simulink model "ps3"  (R2023a)
settings: Solver=ode4  StartTime=0.0  StopTime=t_duration  FixedStep=dt  MaxStep=max_step_size  RelTol=relative_tolerance
values from neighbouring files (symbols this model uses):
  plant = struct()    [ps3_config.m]
settings Model: Creator=ndelurgio  LastModifiedBy=ndelurgio

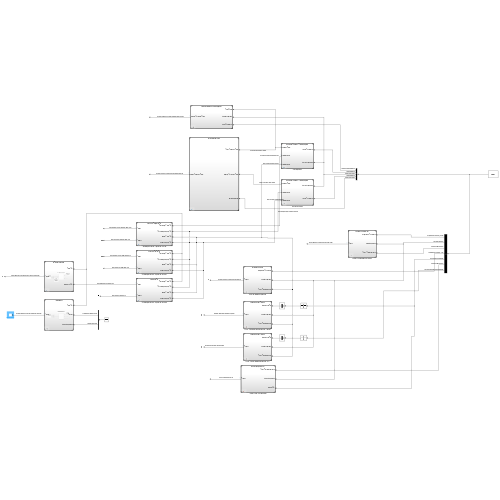
[thumbnail: Simulink's stored preview of the top-level diagram]
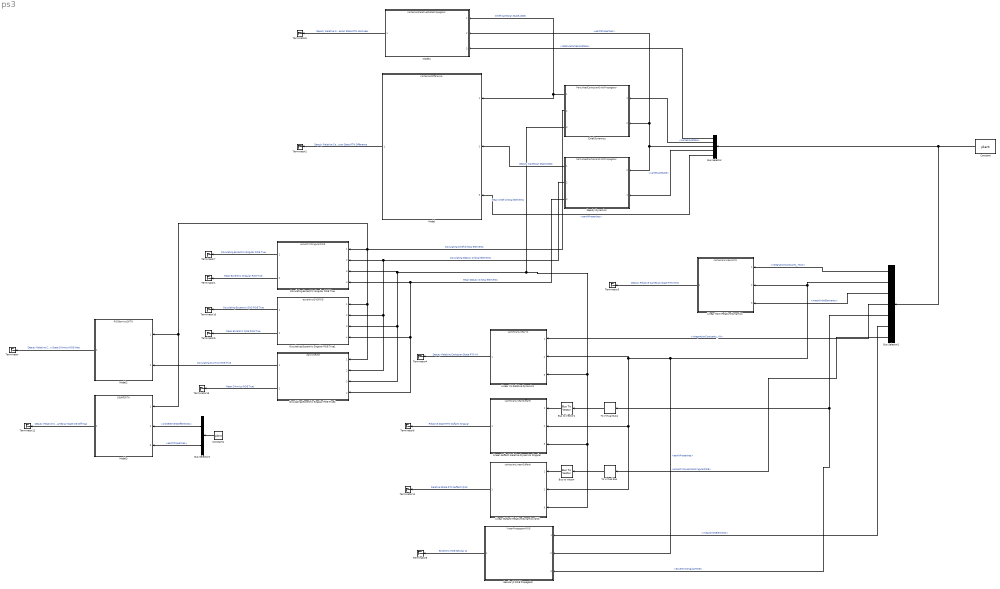
== system ps3 ==
  Bus Selector : BusSelector  OutputSignals=deputy.initialConditions.relativeCartesianState,chief.initialConditions.cartesianState,environment.earthProperties,deputy.initialConditions.cartesianState,environment.earthProperties
  Bus Selector1 : BusSelector  OutputSignals=deputy.initialConditions.integrationConstants_HCW,environment.earthProperties,chief.initialConditions.meanOrbitElements,deputy.initialConditions.integrationConstants_YA,deputy.initialConditions.eccentricSingularROE,chief.initialConditions.meanOrbitElements,deputy.initialConditions.eccentricQuasiNonsingularROE
  Bus Selector2 : BusSelector  OutputSignals=deputy.initialConditions.orbitElementDifferences,environment.earthProperties
  Bus to Vector : BusToVector
  Bus to Vector1 : BusToVector
  Chief Dynamics : ModelReference  ModelNameDialog=PerturbedCartesianOrbitPropagator.slx  SimulationMode=Normal  ModelReferenceVersion=1.136
  Constant : Constant  Value=plant  OutDataTypeStr=Bus: plantBus
  Constant1 : Constant  Value=plant  OutDataTypeStr=Bus: plantBus
  Deputy Dynamics : ModelReference  ModelNameDialog=PerturbedCartesianOrbitPropagator.slx  SimulationMode=Normal  ModelReferenceVersion=1.136
      settings: PortSchema="{\"entries\":[{\"content\":{\"sides\":[{\"content\":{\"connectorIds\":[\"In2\",\"In1\"]},\"type\":\"ConnectorPlacement.EquallySpacedRectSide\",\"uuid\":\"4c211678-740f-40f0-887b-605a3322d7cb\"},{\"content\":{\"connectorIds\":[\"Out1\",\"Out2\",\"Out3\"],\"side\":\"RIGHT\"},\"type\":\"ConnectorPlacement.EquallySpacedRectSide\",\"uuid\":\"7e8d6e44-a7a2-4633-9eac-45eb2a30ed1c\"},{\"content\":{\"side\":\"TOP\"},\"type\":\"ConnectorPlacement.EquallySpacedRectSide\",\"uuid\":\"00358f8f-509c-447f-b607-9e6e4b9aa7b5\"}]},\"type\":\"ConnectorPlacement.EquallySpacedConnector\",\"uuid\":\"f8258235-53bd-4241-8f5f-7f5c3c0a64eb\"}],\"packageUris\":[\"http://schema.mathworks.com/mf0/Connector/R2020b\"],\"version\":\"1.0\"}"
  Linear Guffanti Relative Dynamics QNS : ModelReference  ModelNameDialog=cartesianLinearGuffanti  SimulationMode=Normal  ModelReferenceVersion=1.29
  Linear Guffanti Relative Dynamics Singular : ModelReference  ModelNameDialog=cartesianLinearGuffanti  SimulationMode=Normal  ModelReferenceVersion=1.29
  Linear HCW Relative Dynamics : ModelReference  ModelNameDialog=cartesianLinearHCW  SimulationMode=Normal  ModelReferenceVersion=1.11
  Linear YA Relative Dynamics : ModelReference  ModelNameDialog=cartesianLinearYA  SimulationMode=Normal  ModelReferenceVersion=1.23
  Model : ModelReference  ModelNameDialog=cartesianDifference  SimulationMode=Normal  ModelReferenceVersion=1.33
  Model1 : ModelReference  ModelNameDialog=cartesianRelativeStatePropagator  SimulationMode=Normal  ModelReferenceVersion=1.41
  Model2 : ModelReference  ModelNameDialog=ROEdamico2RTN  SimulationMode=Normal  ModelReferenceVersion=1.9
  Model3 : ModelReference  ModelNameDialog=OEdiff2RTN  SimulationMode=Normal  ModelReferenceVersion=1.12
  Osculating Eccentric Singular ROE True : ModelReference  ModelNameDialog=eccentricSingularROE  SimulationMode=Normal  ModelReferenceVersion=1.13
  Osculating Eccentric Singular ROE True1 : ModelReference  ModelNameDialog=eccentricQNSROE  SimulationMode=Normal  ModelReferenceVersion=1.16
  Osculating Eccentric Singular ROE True2 : ModelReference  ModelNameDialog=damicoROE  SimulationMode=Normal  ModelReferenceVersion=1.17
  Secular J2 ROE Propagator : ModelReference  ModelNameDialog=linearPropagatorROE  SimulationMode=Normal  ModelReferenceVersion=1.11
  Terminator{,1..13} (14 alike) : Terminator
  To Virtual Bus : SignalConversion  ConversionOutput=Virtual bus  OverrideOpt=off
  To Virtual Bus1 : SignalConversion  ConversionOutput=Virtual bus  OverrideOpt=off
  wires:
  Constant/1 -> Bus Selector/1, Bus Selector1/1
  Bus Selector/3 -> Model1/2, Chief Dynamics/2, Deputy Dynamics/2  "<earthProperties>"
  Bus Selector/2 -> Chief Dynamics/1  "<cartesianState>"
  Bus Selector/4 -> Deputy Dynamics/1  "<cartesianState>"
  Chief Dynamics/1 -> Model/1, Model1/1  "Chief Cartesian State J2000"
  Deputy Dynamics/1 -> Model/2  "Deputy Cartesian State J2000"
  Chief Dynamics/2 -> Osculating Eccentric Singular ROE True2/1, Osculating Eccentric Singular ROE True1/1, Model3/1, Model2/1, Osculating Eccentric Singular ROE True/1  "Osculating Chief Orbital Elements"
  Deputy Dynamics/2 -> Osculating Eccentric Singular ROE True2/2, Osculating Eccentric Singular ROE True1/2, Osculating Eccentric Singular ROE True/2  "Osculating Deputy Orbital Elements"
  Bus Selector/5 -> Model/3  "<earthProperties>"
  Model/1 -> Terminator2/1  "Deputy Relative Cartesian State RTN Difference"
  Bus Selector1/3 -> Linear HCW Relative Dynamics/3  "<meanOrbitElements>"
  Bus Selector1/2 -> Secular J2 ROE Propagator/2, Linear Guffanti Relative Dynamics QNS/2, Linear Guffanti Relative Dynamics Singular/2, Linear YA Relative Dynamics/2, Linear HCW Relative Dynamics/2  "<earthProperties>"
  Bus Selector1/1 -> Linear HCW Relative Dynamics/1  "<integrationConstants_HCW>"
  Linear HCW Relative Dynamics/1 -> Terminator3/1  "Deputy Relative Cartesian State RTN HCW"
  Bus Selector/1 -> Model1/3  "<relativeCartesianState>"
  Linear YA Relative Dynamics/1 -> Terminator4/1  "Deputy Relative Cartesian State RTN YA"
  Bus Selector1/4 -> Linear YA Relative Dynamics/1  "<integrationConstants_YA>"
  Model1/1 -> Terminator5/1  "Deputy Relative Cartesian State RTN Nonlinear"
  Linear Guffanti Relative Dynamics Singular/1 -> Terminator6/1  "Relative State RTN Guffanti Singular"
  Bus Selector1/5 -> Secular J2 ROE Propagator/3, To Virtual Bus1/1  "<eccentricSingularROE>"
  Osculating Eccentric Singular ROE True/1 -> Terminator7/1  "Osculating Eccentric Singular ROE True"
  Secular J2 ROE Propagator/1 -> Terminator8/1  "Eccentric ROE Secular J2"
  Bus Selector1/6 -> Secular J2 ROE Propagator/1  "<meanOrbitElements>"
  Chief Dynamics/3 -> Linear Guffanti Relative Dynamics QNS/3, Linear Guffanti Relative Dynamics Singular/3, Linear YA Relative Dynamics/3, Osculating Eccentric Singular ROE True/3, Osculating Eccentric Singular ROE True2/3, Osculating Eccentric Singular ROE True1/3  "Mean Chief Orbital Elements"
  Deputy Dynamics/3 -> Osculating Eccentric Singular ROE True2/4, Osculating Eccentric Singular ROE True1/4, Osculating Eccentric Singular ROE True/4  "Mean Deputy Orbital Elements"
  Osculating Eccentric Singular ROE True/2 -> Terminator1/1  "Mean Eccentric Singular ROE True"
  Osculating Eccentric Singular ROE True1/1 -> Terminator10/1  "Osculating Eccentric QNS ROE True"
  Osculating Eccentric Singular ROE True1/2 -> Terminator9/1  "Mean Eccentric QNS ROE True"
  Linear Guffanti Relative Dynamics QNS/1 -> Terminator11/1  "Relative State RTN Guffanti QNS"
  Bus Selector1/7 -> To Virtual Bus/1  "<eccentricQuasiNonsingularROE>"
  Bus to Vector/1 -> Linear Guffanti Relative Dynamics QNS/1
  Bus to Vector1/1 -> Linear Guffanti Relative Dynamics Singular/1
  To Virtual Bus/1 -> Bus to Vector/1
  To Virtual Bus1/1 -> Bus to Vector1/1
  Osculating Eccentric Singular ROE True2/1 -> Model2/2  "Osculating D'Amico ROE True"
  Osculating Eccentric Singular ROE True2/2 -> Terminator13/1  "Mean D'Amico ROE True"
  Model2/1 -> Terminator/1  "Deputy Relative Cartesian State D'Amico ROE Map"
  Bus Selector2/2 -> Model3/3  "<earthProperties>"
  Bus Selector2/1 -> Model3/2  "<orbitElementDifferences>"
  Constant1/1 -> Bus Selector2/1
  Model3/1 -> Terminator12/1  "Deputy Relative Cartesian State OE Diff Map"
